simulink model "miniproject3"  (R2021b)
settings: Solver=FixedStepAuto  StartTime=0.0  StopTime=4  FixedStep=0.01  RelTol=1e-3
InitFcn:
  | u20 = 0;
  | R1 = 250;
  | R2 = 9750;
  | C = 220e-6;
  | 
  | b1 = 1/(R1*C);
  | a1c = 1/(((R1*R2)/(R1+R2))*C);
  | a1i = 1/(R2*C);
model workspace (MAT data in the model file):
  C = 0.00022
  R1 = 250
  R1_R2 = 243.75
  R2 = 9750
  x = 1
  x1 = 0
settings Model: Creator=Xavier  LastModifiedBy=Xavier

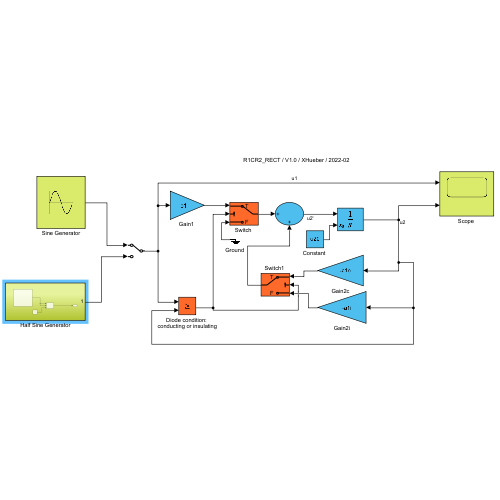
[thumbnail: Simulink's stored preview of the top-level diagram]
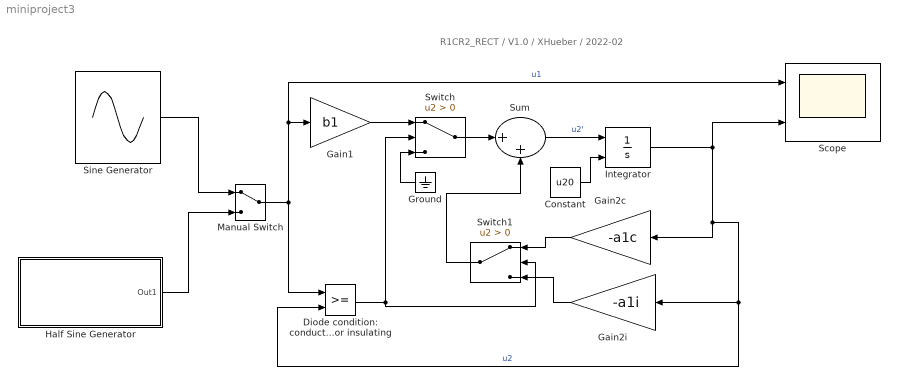
== system miniproject3 ==
  note: R1CR2_RECT / V1.0 / XHueber / 2022-02
  "Constant " : Constant  Value=u20
  Diode condition: conducting or insulating : RelationalOperator  OutDataTypeStr=boolean  RndMeth=Simplest
  "Gain1 " : Gain  Gain=b1
  Gain2c : Gain  Gain=-a1c
  Gain2i : Gain  Gain=-a1i
  "Ground " : Ground
  Half Sine Generator : Subsystem
  Integrator : Integrator  InitialConditionSource=external
  Manual Switch : ManualSwitch
  "Scope " : Scope  NumInputPorts=2
  Sine Generator : Sin  Amplitude=130  Frequency=2*pi  SampleTime=0
  Sum : Sum  Inputs=|++
  "Switch " : Switch  Criteria=u2 > Threshold
  "Switch1 " : Switch  Criteria=u2 > Threshold
  wires:
  Sine Generator/1 -> Manual Switch/1
  Manual Switch/1 -> Diode condition: conducting or insulating/1, "Scope "/1, "Gain1 "/1  "u1"
  "Gain1 "/1 -> "Switch "/1
  Gain2c/1 -> "Switch1 "/1
  Gain2i/1 -> "Switch1 "/3
  Diode condition: conducting or insulating/1 -> "Switch "/2, "Switch1 "/2
  "Switch1 "/1 -> Sum/2
  "Switch "/1 -> Sum/1
  "Ground "/1 -> "Switch "/3
  Sum/1 -> Integrator/1  "u2'"
  "Constant "/1 -> Integrator/2
  Integrator/1 -> "Scope "/2, Gain2c/1, Gain2i/1, Diode condition: conducting or insulating/2  "u2"
  Half Sine Generator/1(Out1) -> Manual Switch/2

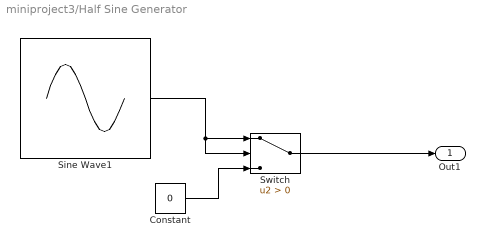
== system miniproject3/Half Sine Generator ==
  Constant : Constant  Value=0
  Sine Wave1 : Sin  Amplitude=130  Frequency=2*pi  SampleTime=0
  Switch : Switch  Criteria=u2 > Threshold
  Out1 : Outport
  wires:
  Sine Wave1/1 -> Switch/2, Switch/1
  Switch/1 -> Out1/1
  Constant/1 -> Switch/3
